simulink model "QAMGainControl"  (R2023a)
settings: Solver=VariableStepAuto  StartTime=0.0  StopTime=tStop  MaxStep=tStepSize  RelTol=1e-3
undefined symbols (not defined in the file): numDelay
libraries: simulink x2
settings Model: Creator=athmajanvivekananthan  LastModifiedBy=athmajanvivekananthan
settings DataIOCC: ReturnWorkspaceOutputs=off

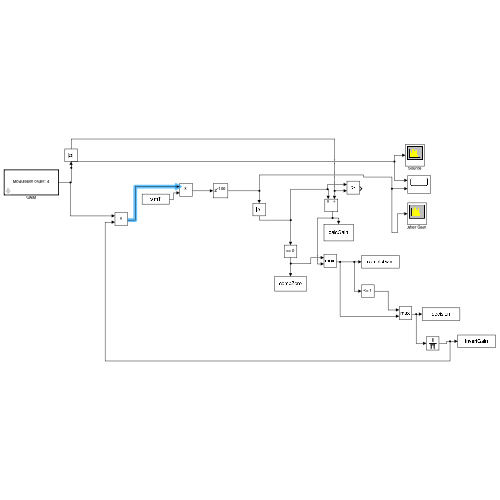
[thumbnail: Simulink's stored preview of the top-level diagram]
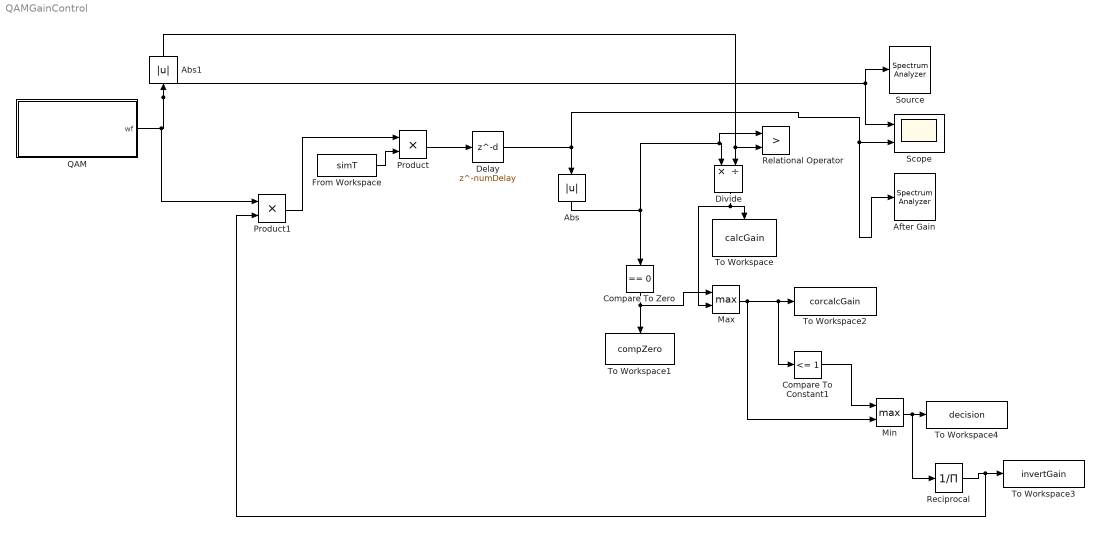
== system QAMGainControl ==
  Abs : Abs  SaturateOnIntegerOverflow=off
  Abs1 : Abs  SaturateOnIntegerOverflow=off
  After Gain : SpectrumAnalyzer  WindowPosition=[35.000000,138.000000,800.000000,500.000000,]  Visible=on  ScopeFrameLocation=window  Span=1000  StartFrequency=-500  StopFrequency=500  YLimits=[-3427.34237515,-2665.71073623]  ColorLimits=[-80 20]
  Compare To Constant1 : simulink/Logic and Bit Operations/Compare To Constant  relop=<=  const=1  OutDataTypeStr=uint8
  Compare To Zero : simulink/Logic and Bit Operations/Compare To Zero  relop===  OutDataTypeStr=uint8
  Delay : Delay  DelayLength=numDelay  InitialCondition=0
  Divide : Product  Inputs=*/
  From Workspace : FromWorkspace  VariableName=simT  OutDataTypeStr=double
  Max : MinMax  Function=max  Inputs=2
  Min : MinMax  Function=max  Inputs=2
  Product : Product
  Product1 : Product
  QAM : MATLAB Function  Tag=BlockGeneratedWWGApp  TreatAsAtomicUnit=on  SystemSampleTime=0.0010000000000000000208  mask(QAM Waveform Generator){nsamps=1, OutputAfterFinalValue=Cyclic repetition}
      mask prompts: nsamps "Samples per frame:"; OutputAfterFinalValue "Form output after final data value by:"
      mask init:
      | %% Generating QAM waveform
      | % QAM configuration
      | M = 4; 	 % Modulation order
      | % input bit source:
      | in = randi([0, 1], 60000, 1);
      | 
      | % Generation
      | waveform = qammod(in, M, 'gray', 'InputType', 'bit', 'UnitAveragePower', true);
      | 
      | Fs = 1000; 								 % Specify the sample rate of the waveform in Hz
      | 
      | %% Configuring block: update parameters and UserData
      | % Get current block
      | thisBlock = gcb;
      | 
      | % Set info parameters
      | maskHandle = Simulink.Mask.get(thisBlock);
      | textFsDialog = maskHandle.getDialogControl('textFs');
      | textFsDialog.Prompt = ['Waveform sample rate (Fs): ' num2str(Fs*1e-6,'%.9g') ' MHz'];
      | textWfLengthDialog = maskHandle.getDialogControl('textWFLength');
      | textWfLengthDialog.Prompt = ['Waveform length: ' num2str(length(waveform)) ' samples'];
      | 
      | % Set sample time of the block
      | set_param(thisBlock, 'SystemSampleTime', num2str(nsamps/Fs,'%.20g'));
      | 
      | % Update UserData
      | cfg.M = M;
      | cfg.Input = in;
      | outVar.WaveformConfig = cfg;
      | outVar.WaveformLength = length(waveform);
      | outVar.Fs = Fs;
      | set_param(thisBlock, 'UserData', outVar);
  Reciprocal : Product  Inputs=/
  Relational Operator : RelationalOperator  Operator=>  OutDataTypeStr=boolean  RndMeth=Simplest  InputSameDT=off
  Scope : Scope  NumInputPorts=2
  Source : SpectrumAnalyzer  WindowPosition=[89.000000,144.000000,800.000000,500.000000,]  Visible=on  ScopeFrameLocation=window  Span=1000  StartFrequency=-500  StopFrequency=500  YLimits=[-6.00356089,3.65468286]  ColorLimits=[-80 20]
  To Workspace : ToWorkspace  VariableName=calcGain  SaveFormat=Timeseries  SampleTime=-1
      settings: Save2DSignal=2-D array (concatenate along first dimension)
  To Workspace1 : ToWorkspace  VariableName=compZero  SaveFormat=Timeseries  SampleTime=-1
  To Workspace2 : ToWorkspace  VariableName=corcalcGain  SaveFormat=Timeseries  SampleTime=-1
  To Workspace3 : ToWorkspace  VariableName=invertGain  SaveFormat=Timeseries  SampleTime=-1
  To Workspace4 : ToWorkspace  VariableName=decision  SaveFormat=Timeseries  SampleTime=-1
  wires:
  From Workspace/1 -> Product/2
  Product/1 -> Delay/1
  Abs1/1 -> Relational Operator/2, Divide/2
  Delay/1 -> Abs/1, Scope/2, After Gain/1
  Divide/1 -> To Workspace/1, Max/2
  Abs/1 -> Compare To Zero/1, Relational Operator/1, Divide/1
  QAM/1(wf) -> Product1/1, Abs1/1, Scope/1, Source/1
  Compare To Zero/1 -> Max/1, To Workspace1/1
  Max/1 -> Min/2, Compare To Constant1/1, To Workspace2/1
  Compare To Constant1/1 -> Min/1
  Min/1 -> Reciprocal/1, To Workspace4/1
  Reciprocal/1 -> Product1/2, To Workspace3/1
  Product1/1 -> Product/1

== matlab function QAMGainControl/QAM ==
  data: wf output; waveform parameter; nsamps parameter; OutputAfterFinalValue parameter
function wf = wfGenerator(waveform, nsamps, OutputAfterFinalValue)

% Create persistent variable
persistent src;

% Preallocate output
wf = complex(zeros(nsamps,size(waveform,2)));

if isempty(src)
    % Get action when signal ends
    if OutputAfterFinalValue == 1
        signalEndAction = 'Cyclic repetition';
    else
        signalEndAction = 'Set to zero';
    end
    
    % Initialize persistent dsp.SignalSource to get current frame
    src = dsp.SignalSource(waveform,nsamps,'SignalEndAction',signalEndAction);
end

% Extract current frame
wf(:,:) = src();

end
